simulink model "my_PV_panel_sun_tracking_simulink"  (R2017b)
settings: Solver=VariableStepAuto  StartTime=0.0  StopTime=3600*14  RelTol=1e-3
values from neighbouring files (symbols this model uses):
  J = m/12*(l^2*cos(beta)^2+d^2*sin(beta)^2+w^2)    [panelMotorParams.m]    (also in solar_panel_data_sun_position.mat = 8.6)
  Kd = 5    [panelMotorParams.m]    (also in solar_panel_data_sun_position.mat)
  Kf = 0.07    [panelMotorParams.m]    (also in solar_panel_data_sun_position.mat)
  Kg = 2000    [panelMotorParams.m]    (also in solar_panel_data_sun_position.mat)
  Kt = 0.07    [panelMotorParams.m]    (also in solar_panel_data_sun_position.mat)
  L = 1e-5    (= 1e-05)    [panelMotorParams.m]    (also in solar_panel_data_sun_position.mat)
  Res = 10    [solar_panel_data_sun_position.mat]
libraries: simulink x1
settings Model: Creator=proso  LastModifiedBy=proso
settings DataIOCC: ExternalInput=[sunTime,sunPosition,sunElevation]  LoadExternalInput=on
settings HardwareCC: TargetBitPerPointer=64  TargetBitPerSizeT=64  TargetBitPerPtrDiffT=64  TargetLongLongMode=on  TargetIntDivRoundTo=Zero  TargetEndianess=LittleEndian  TargetWordSize=64  TargetHWDeviceType=MATLAB Host  ProdEqTarget=off
settings RTWCC: SystemTargetFile=rsim.tlc  TemplateMakefile=rsim_default_tmf  Description=Rapid Simulation Target
settings RSimTargetCC: TargetLangStandard=C99 (ISO)  GeneratePreprocessorConditionals=Use local settings

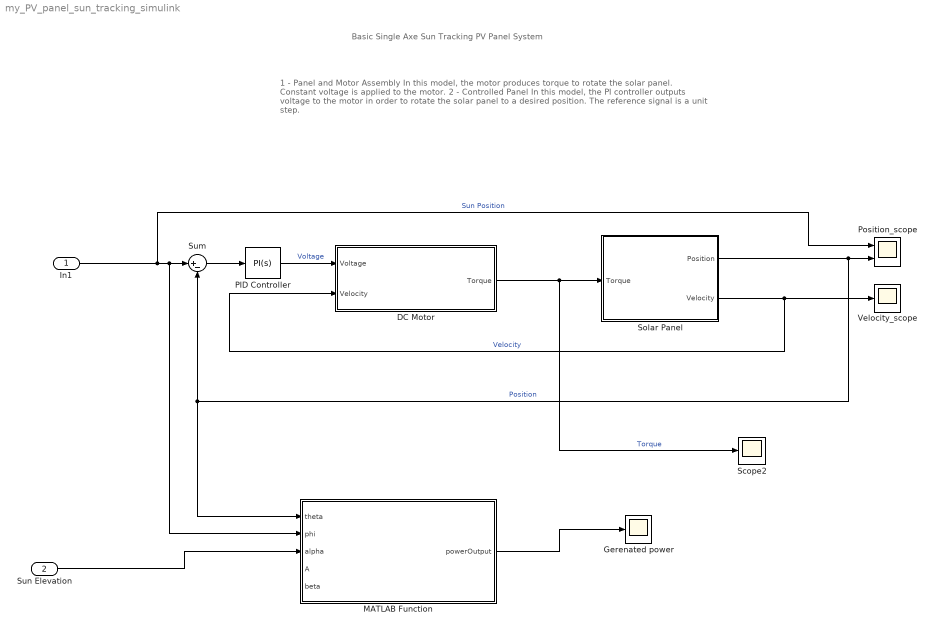
== system my_PV_panel_sun_tracking_simulink ==
  note: 1 - Panel and Motor Assembly
      | In this model, the motor produces torque to rotate the solar panel. Constant voltage is applied to the motor.
      |
      | 2 - Controlled Panel
      | In this model, the PI controller outputs voltage to the motor in order to rotate the solar panel to a desired position. The reference signal is a unit step.
  note: Basic Single Axe Sun Tracking PV Panel System
  In1 : Inport
  Sun Elevation : Inport  Port=2
  DC Motor : Subsystem
  Gerenated power : Scope
  MATLAB Function : MATLAB Function  TreatAsAtomicUnit=on
  PID Controller : simulink/Continuous/PID Controller  Controller=PI  TimeDomain=Continuous-time  SampleTime=-1  IntegratorMethod=Forward Euler  FilterMethod=Forward Euler  Form=Parallel  UseFilter=on  ControllerParametersSource=internal  P=240  I=180  D=0  N=100  InitialConditionSource=internal  InitialConditionForIntegrator=0  InitialConditionForFilter=0  ExternalReset=none  LimitOutput=off  UpperSaturationLimit=inf  LowerSaturationLimit=-inf  LinearizeAsGain=on  AntiWindupMode=none  Kb=1  TrackingMode=off  Kt=1  PParamMin=[]  PParamMax=[]  IParamMin=[]  IParamMax=[]  DParamMin=[]  DParamMax=[]  NParamMin=[]  NParamMax=[]  KbParamMin=[]  KbParamMax=[]  KtParamMin=[]  KtParamMax=[]  POutMin=[]  POutMax=[]  IOutMin=[]  IOutMax=[]  DOutMin=[]  DOutMax=[]  NOutMin=[]  NOutMax=[]  KbOutMin=[]  KbOutMax=[]  KtOutMin=[]  KtOutMax=[]  IntegratorOutMin=[]  IntegratorOutMax=[]  FilterOutMin=[]  FilterOutMax=[]  SumOutMin=[]  SumOutMax=[]  SumI1OutMin=[]  SumI1OutMax=[]  SumI2OutMin=[]  SumI2OutMax=[]  SumI3OutMin=[]  SumI3OutMax=[]  SumDOutMin=[]  SumDOutMax=[]  SaturationOutMin=[]  SaturationOutMax=[]  IntegratorContinuousStateAttributes=''  IntegratorStateMustResolveToSignalObject=off  IntegratorRTWStateStorageClass=Auto  FilterContinuousStateAttributes=''  FilterStateMustResolveToSignalObject=off  FilterRTWStateStorageClass=Auto  DifferentiatorICPrevScaledInput=0  DifferentiatorOutMin=[]  DifferentiatorOutMax=[]  InitialConditionSetting=State (most efficient)  FilterDiffOutCoefMin=[]  FilterDiffOutCoefMax=[]  SumDenOutMin=[]  SumDenOutMax=[]  SumNumOutMin=[]  SumNumOutMax=[]  ReciprocalOutMin=[]  ReciprocalOutMax=[]  DivideOutMin=[]  DivideOutMax=[]  TunerSelectOption=Transfer Function Based (PID Tuner App)
  Position_scope : Scope  NumInputPorts=2
  Scope2 : Scope
  Solar Panel : Subsystem
  Sum : Sum  Inputs=|+-
  Velocity_scope : Scope
  wires:
  Solar Panel/1(Position) -> Position_scope/2, MATLAB Function/1(theta), Sum/2  "Position"
  Solar Panel/2("Velocity ") -> Velocity_scope/1, DC Motor/2(Velocity)  "Velocity"
  PID Controller/1 -> DC Motor/1(Voltage)  "Voltage"
  Sum/1 -> PID Controller/1
  In1/1 -> Position_scope/1, MATLAB Function/2(phi), Sum/1  "Sun Position"
  DC Motor/1(Torque) -> Solar Panel/1(Torque), Scope2/1  "Torque"
  MATLAB Function/1(powerOutput) -> Gerenated power/1
  Sun Elevation/1 -> MATLAB Function/3(alpha)

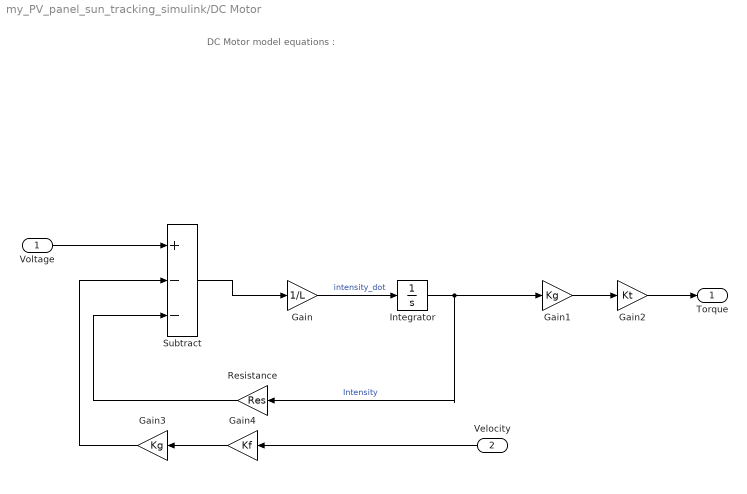
== system my_PV_panel_sun_tracking_simulink/DC Motor ==
  note: DC Motor model equations :
  Voltage : Inport
  Velocity : Inport  Port=2
  Gain : Gain  Gain=1/L
  Gain1 : Gain  Gain=Kg
  Gain2 : Gain  Gain=Kt
  Gain3 : Gain  Gain=Kg
  Gain4 : Gain  Gain=Kf
  Integrator : Integrator
  Resistance : Gain  Gain=Res
  Subtract : Sum  Inputs=+--
  Torque : Outport
  wires:
  Voltage/1 -> Subtract/1
  Resistance/1 -> Subtract/3
  Gain3/1 -> Subtract/2
  Gain4/1 -> Gain3/1
  Gain1/1 -> Gain2/1
  Integrator/1 -> Resistance/1, Gain1/1  "Intensity"
  Gain2/1 -> Torque/1
  Gain/1 -> Integrator/1  "intensity_dot"
  Subtract/1 -> Gain/1
  Velocity/1 -> Gain4/1

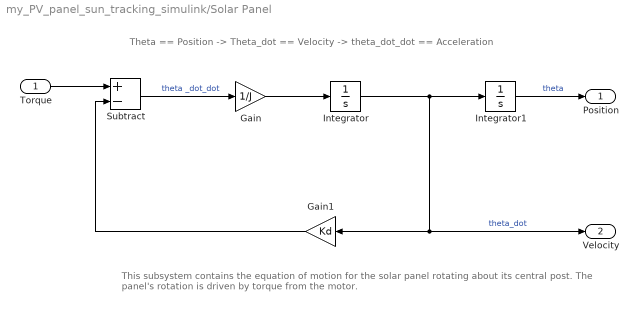
== system my_PV_panel_sun_tracking_simulink/Solar Panel ==
  note: Theta == Position -> Theta_dot == Velocity -> theta_dot_dot == Acceleration
  note: This subsystem contains the equation of motion for the solar panel rotating about its central post.
      | The panel's rotation is driven by torque from the motor.
  Torque : Inport
  Gain : Gain  Gain=1/J
  Gain1 : Gain  Gain=Kd
  Integrator : Integrator
  Integrator1 : Integrator
  Subtract : Sum  Inputs=+-
  Position : Outport
  "Velocity " : Outport  Port=2
  wires:
  Torque/1 -> Subtract/1
  Gain1/1 -> Subtract/2
  Integrator/1 -> Integrator1/1, "Velocity "/1, Gain1/1  "theta_dot"
  Gain/1 -> Integrator/1
  Integrator1/1 -> Position/1  "theta"
  Subtract/1 -> Gain/1  "theta _dot_dot"

== matlab function my_PV_panel_sun_tracking_simulink/MATLAB Function ==
  data: theta input; powerOutput output; phi input; alpha input; A input; beta input
function powerOutput = getGeneratedPower(theta, phi, alpha, A, beta)

A=4
beta=2

% Calculate dot product of the incident sun and panel normal vectors
dot_prod = sin(beta)*sin(pi/2-alpha)*cos(theta-phi) ...
    + cos(beta)*cos(pi/2-alpha);

% Calculate the direct power
powerOutput = 1.353*0.7.^(sin(alpha).^-0.678)*dot_prod*A*0.195*1000; % W

% Replace negative power values with zero (sun is behind the panel)
powerOutput = max(powerOutput,0);
